simulink model "Simulink_Roll_Model_1"  (R2025b)
settings: Solver=VariableStepAuto  StartTime=0.0  StopTime=20  MaxStep=1e-2  RelTol=1e-4
InitFcn:
  | P = parameters_initialise_roll_control();
libraries: simulink_extras x3, aerolibactuator x1
settings Model: Creator=James  LastModifiedBy=James

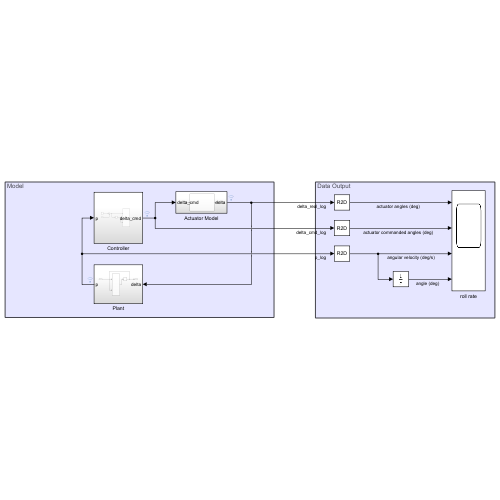
[thumbnail: Simulink's stored preview of the top-level diagram]
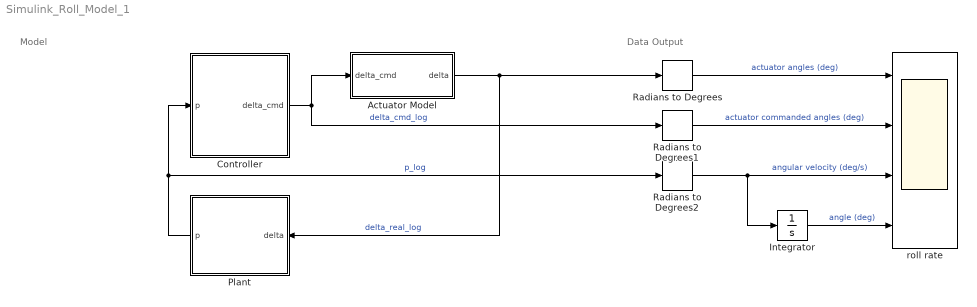
== system Simulink_Roll_Model_1 ==
  note: Model
  note: Data Output
  Actuator Model : Subsystem
  Controller : Subsystem
  Integrator : Integrator
  Plant : Subsystem
  Radians to Degrees : simulink_extras/Transformations/Radians to Degrees
  Radians to Degrees1 : simulink_extras/Transformations/Radians to Degrees
  Radians to Degrees2 : simulink_extras/Transformations/Radians to Degrees
  roll rate : Scope  NumInputPorts=4
      settings: ActiveDisplayYMinimum=2.9392382475235004  ActiveDisplayYMaximum=3.4936110175473938
  wires:
  Controller/1(delta_cmd) -> Actuator Model/1(delta_cmd), Radians to Degrees1/1  "delta_cmd_log"
  Radians to Degrees/1 -> roll rate/1  "actuator angles (deg)"
  Radians to Degrees1/1 -> roll rate/2  "actuator commanded angles (deg)"
  Radians to Degrees2/1 -> Integrator/1, roll rate/3  "angular velocity (deg/s)"
  Integrator/1 -> roll rate/4  "angle (deg)"
  Plant/1(p) -> Radians to Degrees2/1, Controller/1(p)  "p_log"
  Actuator Model/1(delta) -> Radians to Degrees/1, Plant/1(delta)  "delta_real_log"

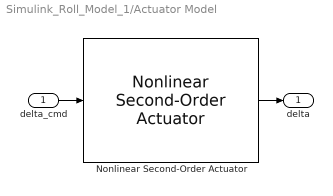
== system Simulink_Roll_Model_1/Actuator Model ==
  delta_cmd : Inport
  Nonlinear Second-Order Actuator : aerolibactuator/Nonlinear Second-Order Actuator  wn_fin=P.Servo.f_N  z_fin=P.Servo.Zeta  fin_max=15*pi/180  fin_min=-15*pi/180  fin_maxrate=P.Servo.Rate  fin_act_0=0  fin_act_vel=0
  delta : Outport
  wires:
  delta_cmd/1 -> Nonlinear Second-Order Actuator/1
  Nonlinear Second-Order Actuator/1 -> delta/1

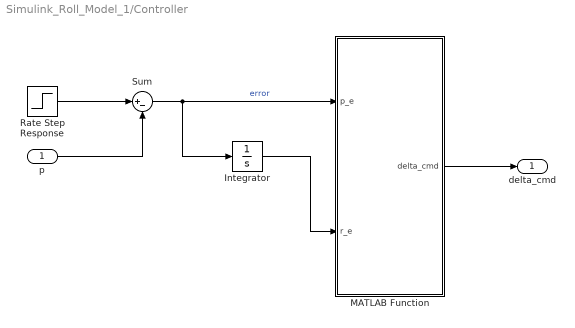
== system Simulink_Roll_Model_1/Controller ==
  p : Inport
  Integrator : Integrator
  MATLAB Function : MATLAB Function  TreatAsAtomicUnit=on
  Rate Step Response : Step  Time=0  After=P.Controller.ref  SampleTime=0
  Sum : Sum  Inputs=|+-
  delta_cmd : Outport
  wires:
  MATLAB Function/1(delta_cmd) -> delta_cmd/1
  Integrator/1 -> MATLAB Function/2(r_e)
  Rate Step Response/1 -> Sum/1
  p/1 -> Sum/2
  Sum/1 -> MATLAB Function/1(p_e), Integrator/1  "error"

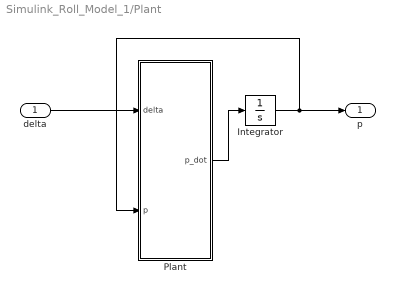
== system Simulink_Roll_Model_1/Plant ==
  delta : Inport
  Integrator : Integrator
  Plant : MATLAB Function  TreatAsAtomicUnit=on
  p : Outport
  wires:
  delta/1 -> Plant/1(delta)
  Integrator/1 -> Plant/2(p), p/1
  Plant/1(p_dot) -> Integrator/1

== matlab function Simulink_Roll_Model_1/Controller/MATLAB Function ==
  data: delta_cmd output; p_e input; r_e input; P parameter
function delta_cmd = controller(p_e, r_e, P)

c = P.Controller.c; %= 150; %Kp gain parameter
Ti = P.Controller.Ti; %= 0.1; %Ki gain parameter
q_e = P.Controller.q_e; % dynamic pressure / pa

Ti = 1/Ti;

Kp = c/q_e;
Ki = Kp/Ti;

delta_cmd = (p_e*Kp) + (r_e*Ki);

== matlab function Simulink_Roll_Model_1/Plant/Plant ==
  data: delta input; p input; p_dot output; P parameter
function p_dot= plant(delta, p, P)

V = P.Vehicle.V;      % Airspeed / m/s
Cl_0 = P.Aero.Cl_0;    % 0 delta Cl
q = P.Aero.q;       % Dynamic Pressure / Pa
d = P.Vehicle.d;       %= 0.062; %Body Diameter / m
Ixx = P.Vehicle.Ixx;     %= 0.00061; %Inertia
s = P.Vehicle.s;       %= 0.02; %Exposed Semi-Span / m
C_r = P.Vehicle.C_r;     %= 0.044; %Root Chord / m
C_t = P.Vehicle.C_t;     %= 0.02; %Tip Chord / m
N = P.Vehicle.N;       %= 4; %Number of canards
C_f = P.Aero.C_f;     %= 0.003; %Flat-plate friction coefficient for body tube
L = P.Vehicle.L;       %= 0.8; %Body Length / m
y_Cp = P.Aero.y_Cp;    %= 0.0315; %Canard radial moment arm / m

S_c     = (C_r + C_t) * s * 0.5; %Canard Area / m^2
AR      = s^2/S_c; %Exposed Aspect Ratio
r       = d/2; %Body Radius / m
A       = pi * r^2; %Area / m^2
mach    = V / 343; %Mach

beta        = sqrt(1 - mach^2); %Prandtl-Glauert
a           = 2*pi*AR / (2 + sqrt(4 + (AR*beta)^2)); %subsonic (Barrowman)
K_fb        = 1 + r/(s + r); %Barrowman Interference Factor ~1.2-1.4
Cl_delta    = K_fb * N * a * (S_c / A) * (y_Cp / d); %Control Effectiveness
 

k               = (C_t - C_r) / s;
I3              = ((r+s)^3 - r^3)/3;
I4              = ((r+s)^4 - r^4)/4;
span_int        = C_r*I3 + k*(I4 - r*I3);

Cl_p_canards    = -2 * K_fb * N * a * span_int / (A * d^2); %Damping
Cl_p_body = -2 * C_f * (L/d);

Cl_p = Cl_p_body + Cl_p_canards;


M_ctrl      = q * A * d * Cl_delta * delta;
M_damp      = (q * A * d^2 * Cl_p * p) / (2*V);
M_dist      = q * A * d * Cl_0;

p_dot = (M_ctrl + M_damp + M_dist) / Ixx;

fprintf('Cl_delta', Cl_delta);
disp(Cl_delta);
fprintf('Cl_p', Cl_p);
disp(Cl_p);
